simulink model "TCS_SLX_FE4"  (R2017a)
settings: Solver=ode45  StartTime=0  StopTime=45  FixedStep=0.001  RelTol=1e-3  AbsTol=1e-6
libraries: Solver_SF x1, simulink x1
settings Model: ExtModeTrigMode=oneshot  ExtModeArmWhenConnect=off  Creator=jhu  LastModifiedBy=Ping
settings DataIOCC: SaveFormat=Array  SignalLoggingSaveFormat=ModelDataLogs  SignalLoggingName=sigsOut
settings OptimizationCC: BlockReduction=off  BooleanDataType=off  ExpressionDepthLimit=2147483647  LifeSpan=inf
settings DebuggingCC: SaveWithParameterizedLinksMsg=none  UnderspecifiedInitializationDetection=Classic  MergeDetectMultiDrivingBlocksExec=none  SignalResolutionControl=TryResolveAllWithWarning  MultiTaskDSMMsg=warning  MultiTaskCondExecSysMsg=none  FcnCallInpInsideContextMsg=warning  StateNameClashWarn=warning  SFUnexpectedBacktrackingDiag=warning  SFNoUnconditionalDefaultTransitionDiag=warning  SFExecutionAtInitializationDiag=none
settings HardwareCC: ProdBitPerPointer=32  ProdBitPerSizeT=32  ProdBitPerPtrDiffT=32  ProdLargestAtomicFloat=None  ProdIntDivRoundTo=Undefined  ProdEndianess=Unspecified  ProdWordSize=32  ProdHWDeviceType=32-bit Generic  TargetUnknown=on
settings ModelReferenceCC: PropagateSignalLabelsOutOfModel=off
settings RTWCC: TemplateMakefile=grt_vc.tmf
settings GRTTargetCC: TargetFcnLib=ansi_tfl_tmw.mat  TargetLangStandard=C89/C90 (ANSI)  GeneratePreprocessorConditionals=Disable all  CombineOutputUpdateFcns=off  GRTInterface=on
settings ConfigComp: CovMetricSettings=dw  CovHtmlReporting=on  CovSaveCumulativeToWorkspaceVar=on  CovSaveSingleToWorkspaceVar=on  CovExternalEMLEnable=off

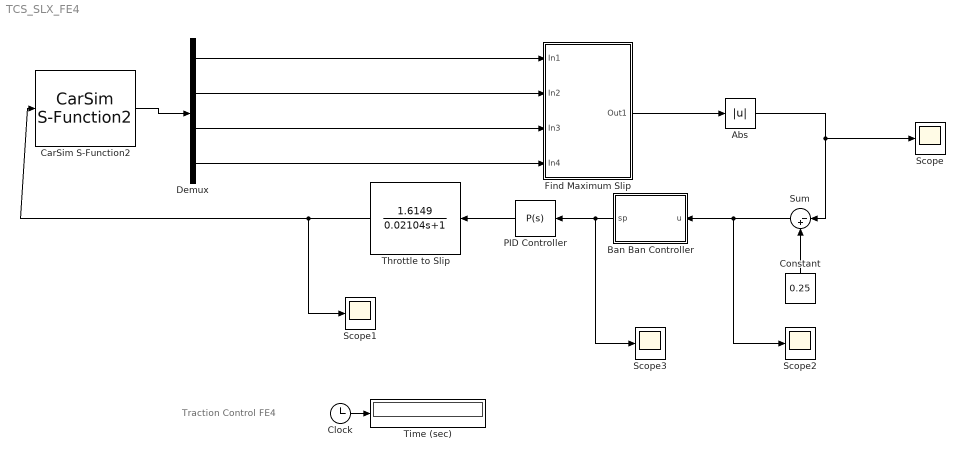
== system TCS_SLX_FE4 ==
  note: Traction Control FE4
  Abs : Abs
  Ban Ban Controller : MATLAB Function  TreatAsAtomicUnit=on
  CarSim S-Function2 : Solver_SF/CarSim S-Function2  Priority=1  VehicleCode=i_i  SIMFILE=simfile.sim
      settings: AttributesFormatString=Vehicle Code: %<VehicleCode>
  Clock : Clock
  Constant : Constant  Value=0.25
  Demux : Demux
  Find Maximum Slip : Subsystem
  PID Controller : simulink/Continuous/PID Controller  Controller=P  TimeDomain=Continuous-time  SampleTime=-1  IntegratorMethod=Forward Euler  FilterMethod=Forward Euler  Form=Parallel  UseFilter=on  ControllerParametersSource=internal  P=5  I=1  D=0  N=100  InitialConditionSource=internal  InitialConditionForIntegrator=0  InitialConditionForFilter=0  ExternalReset=none  LimitOutput=off  UpperSaturationLimit=inf  LowerSaturationLimit=-inf  LinearizeAsGain=on  AntiWindupMode=none  Kb=1  TrackingMode=off  Kt=1  PParamMin=[]  PParamMax=[]  IParamMin=[]  IParamMax=[]  DParamMin=[]  DParamMax=[]  NParamMin=[]  NParamMax=[]  KbParamMin=[]  KbParamMax=[]  KtParamMin=[]  KtParamMax=[]  POutMin=[]  POutMax=[]  IOutMin=[]  IOutMax=[]  DOutMin=[]  DOutMax=[]  NOutMin=[]  NOutMax=[]  KbOutMin=[]  KbOutMax=[]  KtOutMin=[]  KtOutMax=[]  IntegratorOutMin=[]  IntegratorOutMax=[]  FilterOutMin=[]  FilterOutMax=[]  SumOutMin=[]  SumOutMax=[]  SumI1OutMin=[]  SumI1OutMax=[]  SumI2OutMin=[]  SumI2OutMax=[]  SumI3OutMin=[]  SumI3OutMax=[]  SumDOutMin=[]  SumDOutMax=[]  SaturationOutMin=[]  SaturationOutMax=[]  IntegratorContinuousStateAttributes=''  IntegratorStateMustResolveToSignalObject=off  IntegratorRTWStateStorageClass=Auto  FilterContinuousStateAttributes=''  FilterStateMustResolveToSignalObject=off  FilterRTWStateStorageClass=Auto  DifferentiatorICPrevScaledInput=0  DifferentiatorOutMin=[]  DifferentiatorOutMax=[]  InitialConditionSetting=State (most efficient)
  Scope{,1..3} (4 alike) : Scope
  Sum : Sum  Inputs=|-+
  Throttle to Slip : TransferFcn  Numerator=[1.6149]  Denominator=[0.02104 1]
  Time (sec) : Display
      settings: Format=bank  Decimation=100
  wires:
  Clock/1 -> Time (sec)/1
  CarSim S-Function2/1 -> Demux/1
  Demux/1 -> Find Maximum Slip/1(In1)
  Demux/2 -> Find Maximum Slip/2(In2)
  Demux/3 -> Find Maximum Slip/3(In3)
  Demux/4 -> Find Maximum Slip/4(In4)
  Find Maximum Slip/1(Out1) -> Abs/1
  Constant/1 -> Sum/2
  Sum/1 -> Scope2/1, Ban Ban Controller/1(u)
  Ban Ban Controller/1(sp) -> Scope3/1, PID Controller/1
  PID Controller/1 -> Throttle to Slip/1
  Throttle to Slip/1 -> Scope1/1, CarSim S-Function2/1
  Abs/1 -> Scope/1, Sum/1

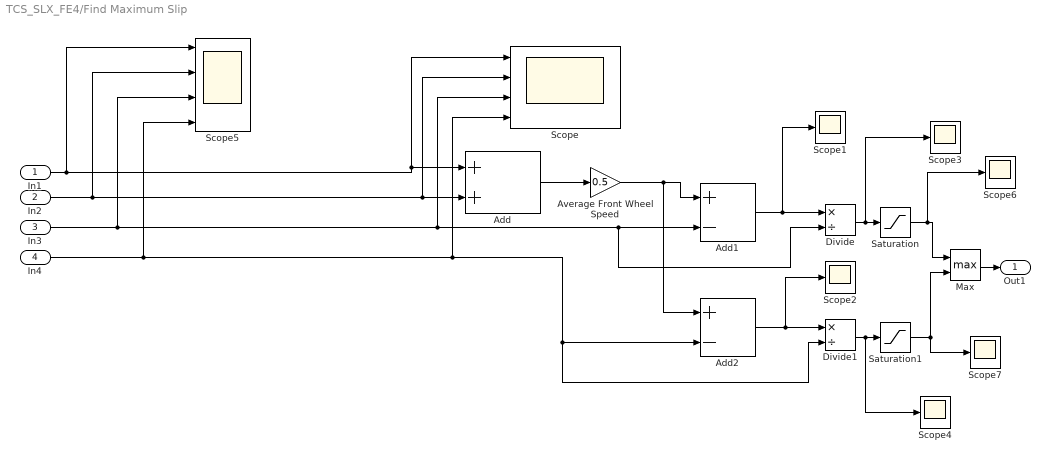
== system TCS_SLX_FE4/Find Maximum Slip ==
  In1 : Inport
  In2 : Inport  Port=2
  In3 : Inport  Port=3
  In4 : Inport  Port=4
  Add : Sum
  Add1 : Sum  Inputs=+-
  Add2 : Sum  Inputs=+-
  Average Front Wheel Speed : Gain  Gain=0.5
  Divide : Product  Inputs=*/  OutMin=[0]  OutMax=[1]
  Divide1 : Product  Inputs=*/  OutMin=[0]  OutMax=[1]
  Max : MinMax  Function=max  Inputs=2
  Saturation : Saturate  UpperLimit=1  LowerLimit=0
  Saturation1 : Saturate  UpperLimit=1  LowerLimit=0
  Scope : Scope  NumInputPorts=4
  Scope{1..4,6..7} (6 alike) : Scope
  Scope5 : Scope  NumInputPorts=4
  Out1 : Outport
  wires:
  Max/1 -> Out1/1
  Add/1 -> Average Front Wheel Speed/1
  Add2/1 -> Scope2/1, Divide1/1
  Average Front Wheel Speed/1 -> Add2/1, Add1/1
  Divide/1 -> Scope3/1, Saturation/1
  Saturation/1 -> Scope6/1, Max/1
  Divide1/1 -> Saturation1/1, Scope4/1
  Saturation1/1 -> Scope7/1, Max/2
  Add1/1 -> Scope1/1, Divide/1
  In4/1 -> Scope/4, Divide1/2, Add2/2, Scope5/4
  In3/1 -> Scope/3, Divide/2, Add1/2, Scope5/3
  In2/1 -> Scope/2, Add/2, Scope5/2
  In1/1 -> Scope/1, Add/1, Scope5/1

== matlab function TCS_SLX_FE4/Ban Ban Controller ==
  data: u input; sp output
function sp = fcn(u)
%Only active while slip signal is negtive 
if u<0
    u_1 = u;
else 
    u_1 = 0;
end

sp = u_1;
